simulink model "All_Simulations"  (R2022b)
settings: Solver=VariableStepAuto  StartTime=0.0  StopTime=10  FixedStep=1e-5  RelTol=1e-3
values from neighbouring files (symbols this model uses):
  A_e = double(subs(A, [q1, q2, q3, dq1, dq2, dq3, tau1, tau2, tau3], [q1_e, q2_e, q3_e, dq1_e, dq2_e, dq3_e, tau1_e, tau2_e, tau3_e]))    [Linearization_SS_Control.m]
  B_e = double(subs(B, [q1, q2, q3, dq1, dq2, dq3, tau1, tau2, tau3], [q1_e, q2_e, q3_e, dq1_e, dq2_e, dq3_e, tau1_e, tau2_e, tau3_e]))    [Linearization_SS_Control.m]
  C_e = [1 0 0 0 0 0; 0 1 0 0 0 0; 0 0 1 0 0 0]    [Linearization_SS_Control.m]
  L = -inv(C_e*inv(A_e-B_e*K)*B_e)    [Linearization_SS_Control.m]
undefined symbols (not defined in the file or in its folder): K
settings Model: Creator=User  LastModifiedBy=User
settings DataIOCC: ReturnWorkspaceOutputs=off

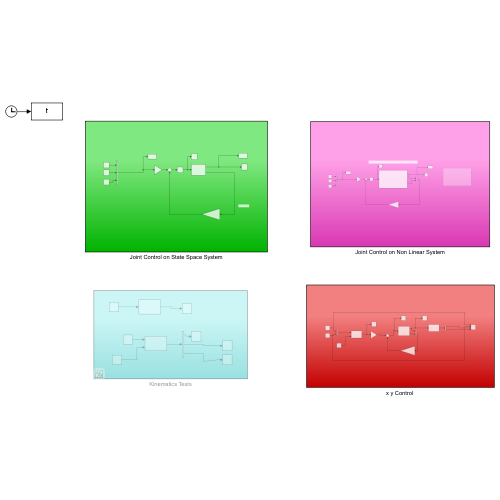
[thumbnail: Simulink's stored preview of the top-level diagram]
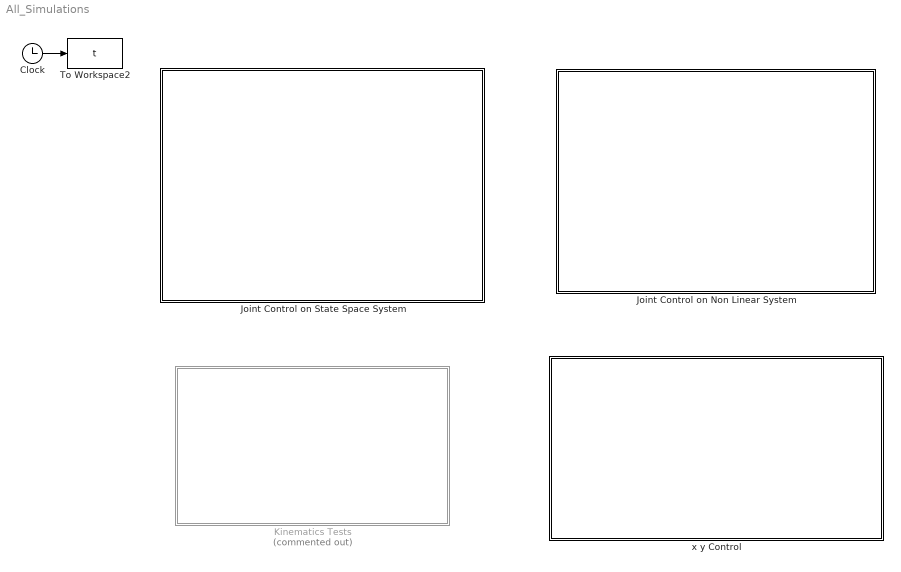
== system All_Simulations ==
  Clock : Clock
  Joint Control on Non Linear System : Subsystem
  Joint Control on State Space System : Subsystem
  Kinematics Tests : Subsystem  Commented=on
  To Workspace2 : ToWorkspace  VariableName=t  SampleTime=-1
  "x y Control " : Subsystem
  wires:
  Clock/1 -> To Workspace2/1

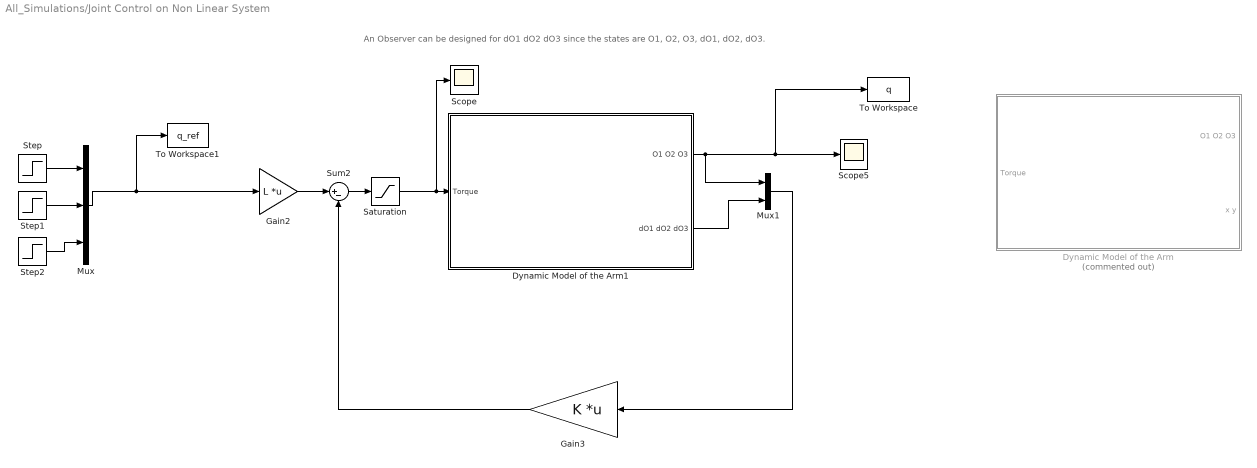
== system All_Simulations/Joint Control on Non Linear System ==
  note: An Observer can be designed for dO1 dO2 dO3 since the states are O1, O2, O3, dO1, dO2, dO3.
  Dynamic Model of the Arm : Subsystem  Commented=on
  Dynamic Model of the Arm1 : Subsystem
  Gain2 : Gain  Gain=L  Multiplication=Matrix(K*u)
  Gain3 : Gain  Gain=K  Multiplication=Matrix(K*u)
  Mux : Mux  Inputs=3
  Mux1 : Mux  Inputs=2
  Saturation : Saturate  UpperLimit=3  LowerLimit=0
  Scope : Scope
  Scope5 : Scope
  Step : Step  Time=0  After=0.2  SampleTime=0
  Step1 : Step  Time=0  After=0  SampleTime=0
  Step2 : Step  Time=0  After=0.5  SampleTime=0
  Sum2 : Sum  Inputs=|+-
  To Workspace : ToWorkspace  VariableName=q  SampleTime=-1
  To Workspace1 : ToWorkspace  VariableName=q_ref  SampleTime=-1
  wires:
  Gain2/1 -> Sum2/1
  Mux/1 -> Gain2/1, To Workspace1/1
  Dynamic Model of the Arm1/2(dO1 dO2 dO3) -> Mux1/2
  Gain3/1 -> Sum2/2
  Mux1/1 -> Gain3/1
  Sum2/1 -> Saturation/1
  Saturation/1 -> Scope/1, Dynamic Model of the Arm1/1(Torque)
  Step/1 -> Mux/1
  Step1/1 -> Mux/2
  Step2/1 -> Mux/3
  Dynamic Model of the Arm1/1(O1 O2 O3) -> To Workspace/1, Scope5/1, Mux1/1

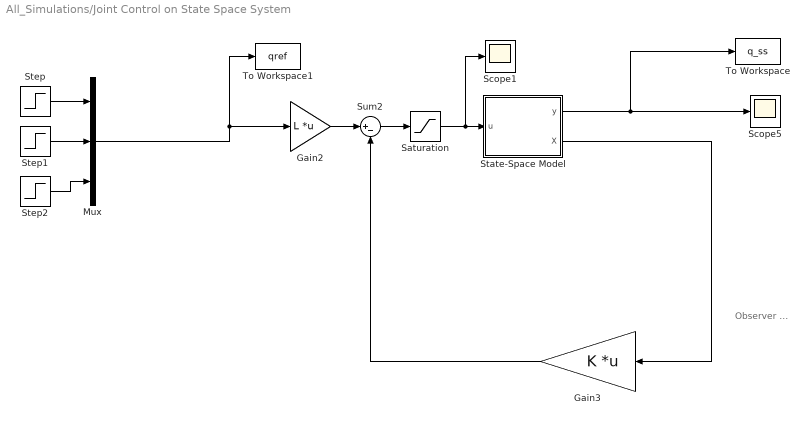
== system All_Simulations/Joint Control on State Space System ==
  note: Observer ...
  Gain2 : Gain  Gain=L  Multiplication=Matrix(K*u)
  Gain3 : Gain  Gain=K  Multiplication=Matrix(K*u)
  Mux : Mux  Inputs=3
  Saturation : Saturate  UpperLimit=3  LowerLimit=-0.01  ZeroCross=off
  Scope1 : Scope
  Scope5 : Scope
  State-Space Model : Subsystem
  Step : Step  Time=0  After=0.2  SampleTime=0
  Step1 : Step  Time=0  After=0  SampleTime=0
  Step2 : Step  Time=0  After=0.5  SampleTime=0
  Sum2 : Sum  Inputs=|+-
  To Workspace : ToWorkspace  VariableName=q_ss  SampleTime=-1
  To Workspace1 : ToWorkspace  VariableName=qref  SampleTime=-1
  wires:
  State-Space Model/2(X) -> Gain3/1
  State-Space Model/1(y) -> To Workspace/1, Scope5/1
  Gain3/1 -> Sum2/2
  Mux/1 -> To Workspace1/1, Gain2/1
  Gain2/1 -> Sum2/1
  Saturation/1 -> Scope1/1, State-Space Model/1(u)
  Sum2/1 -> Saturation/1
  Step/1 -> Mux/1
  Step1/1 -> Mux/2
  Step2/1 -> Mux/3

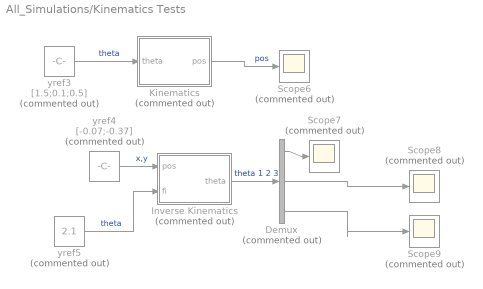
== system All_Simulations/Kinematics Tests ==
  Demux : Demux  Commented=on  Outputs=3
  Inverse Kinematics : MATLAB Function  Commented=on  TreatAsAtomicUnit=on
  Kinematics : MATLAB Function  Commented=on  TreatAsAtomicUnit=on
  Scope{6..9} (4 alike) : Scope  Commented=on
  yref3 : Constant  Commented=on  Value=[1.5;0.1;0.5]
  yref4 : Constant  Commented=on  Value=[-0.07;-0.37]
  yref5 : Constant  Commented=on  Value=2.1
  wires:
  Kinematics/1(pos) -> Scope6/1  "pos"
  yref4/1 -> Inverse Kinematics/1(pos)  "x,y"
  Demux/2 -> Scope8/1
  Inverse Kinematics/1(theta) -> Demux/1  "theta 1 2 3"
  Demux/3 -> Scope9/1
  yref3/1 -> Kinematics/1(theta)  "theta"
  yref5/1 -> Inverse Kinematics/2(fi)  "theta"
  Demux/1 -> Scope7/1

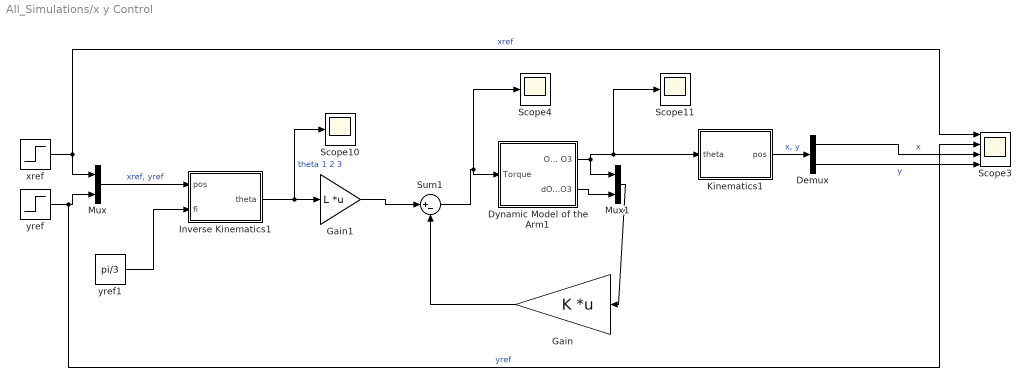
== system All_Simulations/x y Control  ==
  Demux : Demux  Outputs=2
  Dynamic Model of the Arm1 : Subsystem
  Gain : Gain  Gain=K  Multiplication=Matrix(K*u)
  Gain1 : Gain  Gain=L  Multiplication=Matrix(K*u)
  Inverse Kinematics1 : MATLAB Function  TreatAsAtomicUnit=on
  Kinematics1 : MATLAB Function  TreatAsAtomicUnit=on
  Mux : Mux  Inputs=2
  Mux1 : Mux  Inputs=2
  Scope10 : Scope
  Scope11 : Scope
  Scope3 : Scope  NumInputPorts=4
  Scope4 : Scope
  Sum1 : Sum  Inputs=|+-
  xref : Step  Time=0  After=0.1  SampleTime=0
  yref : Step  Time=0  After=0.2  SampleTime=0
  yref1 : Constant  Value=pi/3
  wires:
  Inverse Kinematics1/1(theta) -> Scope10/1, Gain1/1  "theta 1 2 3"
  Sum1/1 -> Dynamic Model of the Arm1/1(Torque), Scope4/1
  Gain/1 -> Sum1/2
  Dynamic Model of the Arm1/1(O1 O2 O3) -> Scope11/1, Kinematics1/1(theta), Mux1/1
  yref1/1 -> Inverse Kinematics1/2(fi)
  Gain1/1 -> Sum1/1
  xref/1 -> Scope3/1, Mux/1  "xref"
  yref/1 -> Scope3/2, Mux/2  "yref"
  Mux/1 -> Inverse Kinematics1/1(pos)  "xref, yref"
  Kinematics1/1(pos) -> Demux/1  "x, y"
  Demux/1 -> Scope3/3  "x"
  Demux/2 -> Scope3/4  "y"
  Dynamic Model of the Arm1/2(dO1 dO2 dO3) -> Mux1/2
  Mux1/1 -> Gain/1

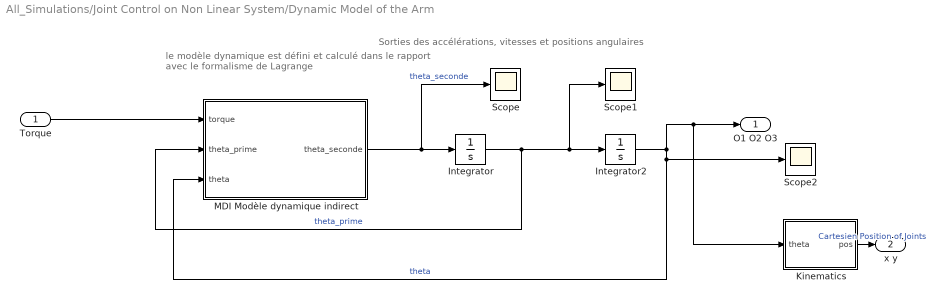
== system All_Simulations/Joint Control on Non Linear System/Dynamic Model of the Arm ==
  note: Sorties des accélérations, vitesses et positions angulaires
  note: le modèle dynamique est défini et calculé dans le rapport avec le formalisme de Lagrange
  Torque : Inport
  Integrator : Integrator  InitialCondition=zeros(3,1)
  Integrator2 : Integrator  InitialCondition=zeros(3,1)
  Kinematics : MATLAB Function  TreatAsAtomicUnit=on
  MDI Modèle dynamique indirect : MATLAB Function  TreatAsAtomicUnit=on
  Scope : Scope
  Scope1 : Scope
  Scope2 : Scope
  O1 O2 O3 : Outport
  x y : Outport  Port=2
  wires:
  MDI Modèle dynamique indirect/1(theta_seconde) -> Scope/1, Integrator/1  "theta_seconde"
  Integrator/1 -> Integrator2/1, Scope1/1, MDI Modèle dynamique indirect/2(theta_prime)  "theta_prime"
  Torque/1 -> MDI Modèle dynamique indirect/1(torque)
  Integrator2/1 -> Scope2/1, MDI Modèle dynamique indirect/3(theta), Kinematics/1(theta), O1 O2 O3/1  "theta"
  Kinematics/1(pos) -> x y/1  "Cartesien Position of Joints"

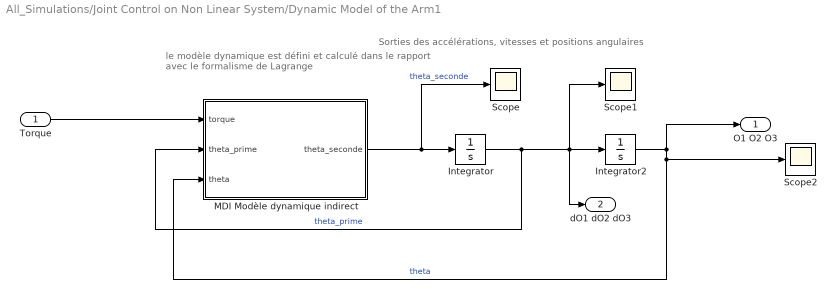
== system All_Simulations/Joint Control on Non Linear System/Dynamic Model of the Arm1 ==
  note: Sorties des accélérations, vitesses et positions angulaires
  note: le modèle dynamique est défini et calculé dans le rapport avec le formalisme de Lagrange
  Torque : Inport
  Integrator : Integrator  InitialCondition=zeros(3,1)
  Integrator2 : Integrator  InitialCondition=zeros(3,1)
  MDI Modèle dynamique indirect : MATLAB Function  TreatAsAtomicUnit=on
  Scope : Scope
  Scope1 : Scope
  Scope2 : Scope
  O1 O2 O3 : Outport
  dO1 dO2 dO3 : Outport  Port=2
  wires:
  MDI Modèle dynamique indirect/1(theta_seconde) -> Scope/1, Integrator/1  "theta_seconde"
  Integrator/1 -> dO1 dO2 dO3/1, Integrator2/1, Scope1/1, MDI Modèle dynamique indirect/2(theta_prime)  "theta_prime"
  Torque/1 -> MDI Modèle dynamique indirect/1(torque)
  Integrator2/1 -> Scope2/1, MDI Modèle dynamique indirect/3(theta), O1 O2 O3/1  "theta"

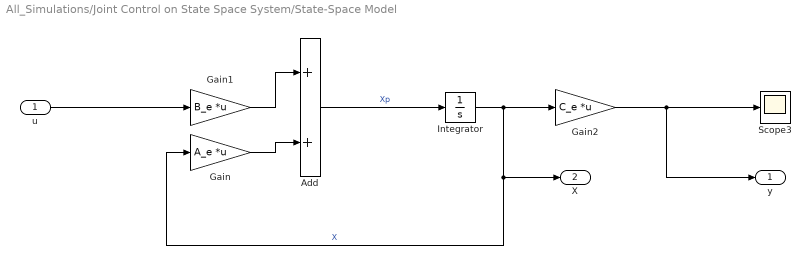
== system All_Simulations/Joint Control on State Space System/State-Space Model ==
  u : Inport
  Add : Sum
  Gain : Gain  Gain=A_e  Multiplication=Matrix(K*u)
  Gain1 : Gain  Gain=B_e  Multiplication=Matrix(K*u)
  Gain2 : Gain  Gain=C_e  Multiplication=Matrix(K*u)
  Integrator : Integrator
  Scope3 : Scope
  y : Outport
  X : Outport  Port=2
  wires:
  Integrator/1 -> Gain2/1, X/1, Gain/1  "X"
  Gain1/1 -> Add/1
  Add/1 -> Integrator/1  "Xp"
  Gain2/1 -> y/1, Scope3/1
  u/1 -> Gain1/1
  Gain/1 -> Add/2

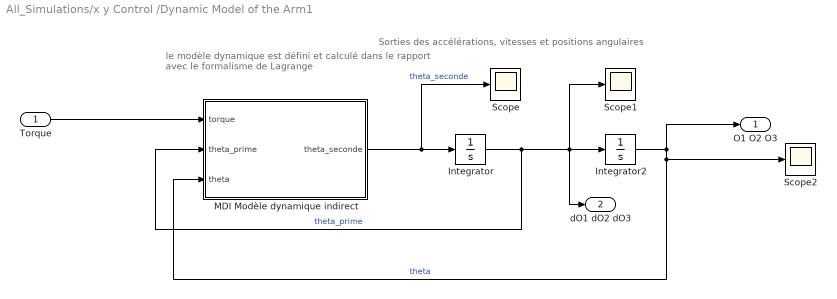
== system All_Simulations/x y Control /Dynamic Model of the Arm1 ==
  note: Sorties des accélérations, vitesses et positions angulaires
  note: le modèle dynamique est défini et calculé dans le rapport avec le formalisme de Lagrange
  Torque : Inport
  Integrator : Integrator  InitialCondition=zeros(3,1)
  Integrator2 : Integrator  InitialCondition=zeros(3,1)
  MDI Modèle dynamique indirect : MATLAB Function  TreatAsAtomicUnit=on
  Scope : Scope
  Scope1 : Scope
  Scope2 : Scope
  O1 O2 O3 : Outport
  dO1 dO2 dO3 : Outport  Port=2
  wires:
  MDI Modèle dynamique indirect/1(theta_seconde) -> Scope/1, Integrator/1  "theta_seconde"
  Integrator/1 -> dO1 dO2 dO3/1, Integrator2/1, Scope1/1, MDI Modèle dynamique indirect/2(theta_prime)  "theta_prime"
  Torque/1 -> MDI Modèle dynamique indirect/1(torque)
  Integrator2/1 -> Scope2/1, MDI Modèle dynamique indirect/3(theta), O1 O2 O3/1  "theta"

== matlab function All_Simulations/Joint Control on Non Linear System/Dynamic Model of the Arm/Kinematics ==
  data: theta input; pos output
function pos= fcn(theta)

% Masses des membres
m1 = 1.3850917e-01; % masse du membre inférieur
m2 = 1.3274562e-01; % masse du membre secondaire
m3 = 1.4327573e-01; % masse de la pince

% Longueurs des membres
l1 = 0.13; % longueur du membre inférieur
l2 = 0.124; % longueur du membre secondaire
l3 = 0.146; % longueur de la pince

theta1 = theta(1);
theta2 = theta(2);
theta3 = theta(3);

x = l1*cos(theta1) + l2*cos(theta1+theta2) + l3*cos(theta1+theta2+theta3);

y = l1*sin(theta1) + l2*sin(theta1+theta2) + l3*sin(theta1+theta2+theta3);


pos = [x ; y];

== matlab function All_Simulations/x y Control /Dynamic Model of the Arm1/MDI Modèle dynamique indirect ==
  data: torque input; theta_seconde output; theta_prime input; theta input
function theta_seconde = mdi(torque, theta_prime, theta)

% Fonction qui traduit le comportement dynamique du robot lors de son mouvement

% Récupération des positions et vitesses angulaires du robot
tp1 = theta_prime(1);
tp2 = theta_prime(2);
tp3 = theta_prime(3);
t1 = theta(1);
t2 = theta(2);
t3 = theta(3);

g = 9.81;

%% Constantes du robot

% Masses des membres
m1 = 1.3850917e-01; % masse du membre inférieur
m2 = 1.3274562e-01; % masse du membre secondaire
m3 = 1.4327573e-01; % masse de la pince

% Longueurs des membres
l1 = 0.13; % longueur du membre inférieur
l2 = 0.124; % longueur du membre secondaire
l3 = 0.146; % longueur de la pince

% lc1 = l1/2;
% lc2 = l2/2;
% lc3 = l3/2;

lc1 = l1;
lc2 = l2;
lc3 = l3;

% Joints Inertia (Taken from Matlab file Inertia_Computation)
I1 = 5.4436e-04; % Kg.m2
I2 = 4.0847e-04; % Kg.m2
I3 = 5.1294e-04; % Kg.m2

%% Calcul de M(theta)




alpha1 = m1*lc1^2 + m2*(l1^2+lc2^2+2*l1*lc2*cos(t2)) + m3*(l1^2+l2^2+lc3^2+2*l1*l2*cos(t2)+2*l2*lc3*cos(t3)+2*l1*lc3*cos(t2+t3));
B = m2*(lc2^2 + l1*lc2*cos(t2)) + m3*(l2^2+lc3^2+l1*l2*cos(t2)+2*l2*lc3*cos(t3)+l1*lc3*cos(t2+t3));
gamma = m3*(lc3^2+l2*lc3*cos(t3)+l1*lc3*cos(t2+t3));
alpha2 = m2*lc2^2+m3*(l2^2+lc3^2+2*l2*lc3*cos(t3));
eta = m3*(lc3^2+l2*lc3*cos(t3));
alpha3 = m3*lc3^2;

M = [ (alpha1 + I1 + I2 + I3) (B + I2 + I3) (gamma + I3) ;
    (B + I2 + I3) (alpha2 + I2 + I3) (eta + I3) ;
    (gamma + I3) (eta + I3) alpha3 + I3 ];


%% Calcul de thetadot . C (theta, thetadot)

% Calcul de M'(teta). tetap

alpha1p = -2*m2*l1*lc2*tp2*sin(t2) -2*m3*l1*l2*tp2*sin(t2) -2*m3*l2*lc3*tp3*sin(t3) -2*m3*l1*lc3*(tp2+tp3)*sin(t2+t3);
Bp = -m2*l1*lc2*tp2*sin(t2) -m3*l1*l2*tp2*sin(t2) -2*m3*l2*lc3*tp3*sin(t3) -m3*l1*lc3*(tp2+tp3)*sin(t2+t3);
gammap = -m3*l2*lc3*tp3*sin(t3) -m3*l1*lc3*(tp2+tp3)*sin(t2+t3);
alpha2p = -2*m3*l2*lc3*tp3*sin(t3) ;
etap = -m3*l2*lc3*tp3*sin(t3) ;
alpha3p = 0;

Mptp = [ tp1*alpha1p + tp2*Bp + tp3*gammap ;
        tp1*Bp + tp2*alpha2p + tp3*etap ;
        tp1*gammap + tp2*etap];



% Calcul de D(teta, tetap)

D = [0;
     -2*m2*l1*lc2*(tp1^2)*sin(t2)-2*m3*l1*l2*(tp1^2)*sin(t2)-2*m3*l1*lc3*(tp1^2)*sin(t2+t3)-2*m2*l1*lc2*tp1*tp2*sin(t2)-2*m3*l1*l2*tp1*tp2*sin(t2)-2*m3*l1*lc3*tp1*tp2*sin(t2+t3)-2*m3*l1*lc3*tp1*tp3*sin(t2+t3);
        -2*m3*l2*lc3*(tp1^2)*sin(t3)-2*m3*l1*lc3*(tp1^2)*sin(t2+t3)-4*m3*l2*lc3*tp1*tp2*sin(t3)-2*m3*l1*lc3*tp1*tp2*sin(t2+t3)-2*m3*l2*lc3*tp1*tp3*sin(t3)-2*m3*l1*lc3*tp1*tp3*sin(t2+t3)-2*m3*l2*lc3*(tp2^2)*sin(t3)-2*m3*l2*lc3*tp2*tp3*sin(t3)];

% Calcul de tetap . C(teta, tetap)

C  = Mptp - 0.5 * D;

%% Calcul de G(teta)

G = [(m1*g*lc1+m2*g*l1+m3*g*l1)*cos(t1)+(m2*g*lc2+m3*g*l2)*cos(t1+t2)+m3*g*lc3*cos(t1+t2+t3) ;
     (m2*g*lc2+m3*g*l2)*cos(t1+t2)+m3*g*lc3*cos(t1+t2+t3);
     m3*g*lc3*cos(t1+t2+t3)];



theta_seconde = inv(M) * (torque - C - G);

== matlab function All_Simulations/Joint Control on Non Linear System/Dynamic Model of the Arm1/MDI Modèle dynamique indirect ==
  data: torque input; theta_seconde output; theta_prime input; theta input
function theta_seconde = mdi(torque, theta_prime, theta)

% Fonction qui traduit le comportement dynamique du robot lors de son mouvement

% Récupération des positions et vitesses angulaires du robot
tp1 = theta_prime(1);
tp2 = theta_prime(2);
tp3 = theta_prime(3);
t1 = theta(1);
t2 = theta(2);
t3 = theta(3);

g = 9.81;

%% Constantes du robot

% Masses des membres
m1 = 1.3850917e-01; % masse du membre inférieur
m2 = 1.3274562e-01; % masse du membre secondaire
m3 = 1.4327573e-01; % masse de la pince

% Longueurs des membres
l1 = 0.13; % longueur du membre inférieur
l2 = 0.124; % longueur du membre secondaire
l3 = 0.146; % longueur de la pince

% lc1 = l1/2;
% lc2 = l2/2;
% lc3 = l3/2;

lc1 = l1;
lc2 = l2;
lc3 = l3;

% Joints Inertia (Taken from Matlab file Inertia_Computation)
I1 = 5.4436e-04; % Kg.m2
I2 = 4.0847e-04; % Kg.m2
I3 = 5.1294e-04; % Kg.m2

%% Calcul de M(theta)




alpha1 = m1*lc1^2 + m2*(l1^2+lc2^2+2*l1*lc2*cos(t2)) + m3*(l1^2+l2^2+lc3^2+2*l1*l2*cos(t2)+2*l2*lc3*cos(t3)+2*l1*lc3*cos(t2+t3));
B = m2*(lc2^2 + l1*lc2*cos(t2)) + m3*(l2^2+lc3^2+l1*l2*cos(t2)+2*l2*lc3*cos(t3)+l1*lc3*cos(t2+t3));
gamma = m3*(lc3^2+l2*lc3*cos(t3)+l1*lc3*cos(t2+t3));
alpha2 = m2*lc2^2+m3*(l2^2+lc3^2+2*l2*lc3*cos(t3));
eta = m3*(lc3^2+l2*lc3*cos(t3));
alpha3 = m3*lc3^2;

M = [ (alpha1 + I1 + I2 + I3) (B + I2 + I3) (gamma + I3) ;
    (B + I2 + I3) (alpha2 + I2 + I3) (eta + I3) ;
    (gamma + I3) (eta + I3) alpha3 + I3 ];


%% Calcul de thetadot . C (theta, thetadot)

% Calcul de M'(teta). tetap

alpha1p = -2*m2*l1*lc2*tp2*sin(t2) -2*m3*l1*l2*tp2*sin(t2) -2*m3*l2*lc3*tp3*sin(t3) -2*m3*l1*lc3*(tp2+tp3)*sin(t2+t3);
Bp = -m2*l1*lc2*tp2*sin(t2) -m3*l1*l2*tp2*sin(t2) -2*m3*l2*lc3*tp3*sin(t3) -m3*l1*lc3*(tp2+tp3)*sin(t2+t3);
gammap = -m3*l2*lc3*tp3*sin(t3) -m3*l1*lc3*(tp2+tp3)*sin(t2+t3);
alpha2p = -2*m3*l2*lc3*tp3*sin(t3) ;
etap = -m3*l2*lc3*tp3*sin(t3) ;
alpha3p = 0;

Mptp = [ tp1*alpha1p + tp2*Bp + tp3*gammap ;
        tp1*Bp + tp2*alpha2p + tp3*etap ;
        tp1*gammap + tp2*etap];



% Calcul de D(teta, tetap)

D = [0;
     -2*m2*l1*lc2*(tp1^2)*sin(t2)-2*m3*l1*l2*(tp1^2)*sin(t2)-2*m3*l1*lc3*(tp1^2)*sin(t2+t3)-2*m2*l1*lc2*tp1*tp2*sin(t2)-2*m3*l1*l2*tp1*tp2*sin(t2)-2*m3*l1*lc3*tp1*tp2*sin(t2+t3)-2*m3*l1*lc3*tp1*tp3*sin(t2+t3);
        -2*m3*l2*lc3*(tp1^2)*sin(t3)-2*m3*l1*lc3*(tp1^2)*sin(t2+t3)-4*m3*l2*lc3*tp1*tp2*sin(t3)-2*m3*l1*lc3*tp1*tp2*sin(t2+t3)-2*m3*l2*lc3*tp1*tp3*sin(t3)-2*m3*l1*lc3*tp1*tp3*sin(t2+t3)-2*m3*l2*lc3*(tp2^2)*sin(t3)-2*m3*l2*lc3*tp2*tp3*sin(t3)];

% Calcul de tetap . C(teta, tetap)

C  = Mptp - 0.5 * D;

%% Calcul de G(teta)

G = [(m1*g*lc1+m2*g*l1+m3*g*l1)*cos(t1)+(m2*g*lc2+m3*g*l2)*cos(t1+t2)+m3*g*lc3*cos(t1+t2+t3) ;
     (m2*g*lc2+m3*g*l2)*cos(t1+t2)+m3*g*lc3*cos(t1+t2+t3);
     m3*g*lc3*cos(t1+t2+t3)];



theta_seconde = inv(M) * (torque - C - G);

== matlab function All_Simulations/Kinematics Tests/Kinematics ==
  data: theta input; pos output
function pos= fcn(theta)

% Masses des membres
m1 = 1.3850917e-01; % masse du membre inférieur
m2 = 1.3274562e-01; % masse du membre secondaire
m3 = 1.4327573e-01; % masse de la pince

% Longueurs des membres
l1 = 0.13; % longueur du membre inférieur
l2 = 0.124; % longueur du membre secondaire
l3 = 0.146; % longueur de la pince

theta1 = theta(1);
theta2 = theta(2);
theta3 = theta(3);

x = l1*cos(theta1) + l2*cos(theta1+theta2) + l3*cos(theta1+theta2+theta3);

y = l1*sin(theta1) + l2*sin(theta1+theta2) + l3*sin(theta1+theta2+theta3);


pos = [x ; y];

== matlab function All_Simulations/Kinematics Tests/Inverse Kinematics ==
  data: pos input; theta output; fi input
function theta= fcn(pos, fi)

% Masses des membres
m1 = 1.3850917e-01; % masse du membre inférieur
m2 = 1.3274562e-01; % masse du membre secondaire
m3 = 1.4327573e-01; % masse de la pince

% Longueurs des membres
l1 = 0.13; % longueur du membre inférieur
l2 = 0.124; % longueur du membre secondaire
l3 = 0.146; % longueur de la pince

x = pos(1);
y = pos(2);


xB = x - l3*cos(fi);
yB = x - l3*sin(fi);

theta2 = acos((xB^2+yB^2-l1^2-l2^2)/(2*l1*l2));

theta1 = asin(((l1+l2*cos(theta2 ))*yB - l2*sin(theta2 )*xB)/(xB^2 +yB^2));

theta3 = fi - theta1 - theta2;


theta = [theta1 ; theta2 ; theta3];

== matlab function All_Simulations/x y Control /Kinematics1 ==
  data: theta input; pos output
function pos= fcn(theta)

% Masses des membres
m1 = 1.3850917e-01; % masse du membre inférieur
m2 = 1.3274562e-01; % masse du membre secondaire
m3 = 1.4327573e-01; % masse de la pince

% Longueurs des membres
l1 = 0.13; % longueur du membre inférieur
l2 = 0.124; % longueur du membre secondaire
l3 = 0.146; % longueur de la pince

theta1 = theta(1);
theta2 = theta(2);
theta3 = theta(3);

x = l1*cos(theta1) + l2*cos(theta1+theta2) + l3*cos(theta1+theta2+theta3);

y = l1*sin(theta1) + l2*sin(theta1+theta2) + l3*sin(theta1+theta2+theta3);


pos = [x ; y];

== matlab function All_Simulations/x y Control /Inverse Kinematics1 ==
  data: pos input; theta output; fi input
function theta= fcn(pos, fi)

% Masses des membres
m1 = 1.3850917e-01; % masse du membre inférieur
m2 = 1.3274562e-01; % masse du membre secondaire
m3 = 1.4327573e-01; % masse de la pince

% Longueurs des membres
l1 = 0.13; % longueur du membre inférieur
l2 = 0.124; % longueur du membre secondaire
l3 = 0.146; % longueur de la pince

x = pos(1);
y = pos(2);


xB = x - l3*cos(fi);
yB = y - l3*sin(fi);

theta2 = acos((xB^2+yB^2-l1^2-l2^2)/(2*l1*l2));

theta1 = asin(((l1+l2*cos(theta2 ))*yB - l2*sin(theta2 )*xB)/(xB^2 +yB^2));

theta3 = fi - theta1 - theta2;


theta = [theta1 ; theta2 ; theta3];

== matlab function All_Simulations/Joint Control on Non Linear System/Dynamic Model of the Arm/MDI Modèle dynamique indirect ==
  data: torque input; theta_seconde output; theta_prime input; theta input
function theta_seconde = mdi(torque, theta_prime, theta)

% Fonction qui traduit le comportement dynamique du robot lors de son mouvement

% Récupération des positions et vitesses angulaires du robot
tp1 = theta_prime(1);
tp2 = theta_prime(2);
tp3 = theta_prime(3);
t1 = theta(1);
t2 = theta(2);
t3 = theta(3);

g = 9.81;

%% Constantes du robot

% Masses des membres
m1 = 1.3850917e-01; % masse du membre inférieur
m2 = 1.3274562e-01; % masse du membre secondaire
m3 = 1.4327573e-01; % masse de la pince

% Longueurs des membres
l1 = 0.13; % longueur du membre inférieur
l2 = 0.124; % longueur du membre secondaire
l3 = 0.146; % longueur de la pince

% lc1 = l1/2;
% lc2 = l2/2;
% lc3 = l3/2;

lc1 = l1;
lc2 = l2;
lc3 = l3;

%I1 = 0.0347563; %kg.m^2
%I2 = 0.0458929; %kg.m^2
%I3 = 0.0347563; %kg.m^2

%% Calcul de M(theta)

% Inertia of links 1, 2 and 3
I1 = (m1*l1^2)/12;
I2 = (m2*l2^2)/12;
I3 = (m3*l3^2)/12;



alpha1 = m1*lc1^2 + m2*(l1^2+lc2^2+2*l1*lc2*cos(t2)) + m3*(l1^2+l2^2+lc3^2+2*l1*l2*cos(t2)+2*l2*lc3*cos(t3)+2*l1*lc3*cos(t2+t3));
B = m2*(lc2^2 + l1*lc2*cos(t2)) + m3*(l2^2+lc3^2+l1*l2*cos(t2)+2*l2*lc3*cos(t3)+l1*lc3*cos(t2+t3));
gamma = m3*(lc3^2+l2*lc3*cos(t3)+l1*lc3*cos(t2+t3));
alpha2 = m2*lc2^2+m3*(l2^2+lc3^2+2*l2*lc3*cos(t3));
eta = m3*(lc3^2+l2*lc3*cos(t3));
alpha3 = m3*lc3^2;

M = [ (alpha1 + I1 + I2 + I3) (B + I2 + I3) (gamma + I3) ;
    (B + I2 + I3) (alpha2 + I2 + I3) (eta + I3) ;
    (gamma + I3) (eta + I3) alpha3 + I3 ];


%% Calcul de thetadot . C (theta, thetadot)

% Calcul de M'(teta). tetap

alpha1p = -2*m2*l1*lc2*tp2*sin(t2) -2*m3*l1*l2*tp2*sin(t2) -2*m3*l2*lc3*tp3*sin(t3) -2*m3*l1*lc3*(tp2+tp3)*sin(t2+t3);
Bp = -m2*l1*lc2*tp2*sin(t2) -m3*l1*l2*tp2*sin(t2) -2*m3*l2*lc3*tp3*sin(t3) -m3*l1*lc3*(tp2+tp3)*sin(t2+t3);
gammap = -m3*l2*lc3*tp3*sin(t3) -m3*l1*lc3*(tp2+tp3)*sin(t2+t3);
alpha2p = -2*m3*l2*lc3*tp3*sin(t3) ;
etap = -m3*l2*lc3*tp3*sin(t3) ;
alpha3p = 0;

Mptp = [ tp1*alpha1p + tp2*Bp + tp3*gammap ;
        tp1*Bp + tp2*alpha2p + tp3*etap ;
        tp1*gammap + tp2*etap];



% Calcul de D(teta, tetap)

D = [0;
     -2*m2*l1*lc2*(tp1^2)*sin(t2)-2*m3*l1*l2*(tp1^2)*sin(t2)-2*m3*l1*lc3*(tp1^2)*sin(t2+t3)-2*m2*l1*lc2*tp1*tp2*sin(t2)-2*m3*l1*l2*tp1*tp2*sin(t2)-2*m3*l1*lc3*tp1*tp2*sin(t2+t3)-2*m3*l1*lc3*tp1*tp3*sin(t2+t3);
        -2*m3*l2*lc3*(tp1^2)*sin(t3)-2*m3*l1*lc3*(tp1^2)*sin(t2+t3)-4*m3*l2*lc3*tp1*tp2*sin(t3)-2*m3*l1*lc3*tp1*tp2*sin(t2+t3)-2*m3*l2*lc3*tp1*tp3*sin(t3)-2*m3*l1*lc3*tp1*tp3*sin(t2+t3)-2*m3*l2*lc3*(tp2^2)*sin(t3)-2*m3*l2*lc3*tp2*tp3*sin(t3)];

% Calcul de tetap . C(teta, tetap)

C  = Mptp - 0.5 * D;

%% Calcul de G(teta)

G = [(m1*g*lc1+m2*g*l1+m3*g*l1)*cos(t1)+(m2*g*lc2+m3*g*l2)*cos(t1+t2)+m3*g*lc3*cos(t1+t2+t3) ;
     (m2*g*lc2+m3*g*l2)*cos(t1+t2)+m3*g*lc3*cos(t1+t2+t3);
     m3*g*lc3*cos(t1+t2+t3)];



theta_seconde = inv(M) * (torque - C - G);
